simulink model "lab4"  (R2015b)
settings: Solver=ode3  StartTime=0  StopTime=30  FixedStep=Ts  RelTol=1e-3
values from neighbouring files (symbols this model uses):
  A = 12.0    (= 12)    [dev_digicomm_lab4.m]
  delta = round(310E-6*fs)    [dev_digicomm_lab4.m]
  poleN = 5    [dev_digicomm_lab4.m]
  pulsPeriod = Tb    (= 0.0003)    [dev_digicomm_lab4.m]
  pulsPhase = Tb/15    (= 2e-05)    [dev_digicomm_lab4.m]
  pulsWidth = 20    [dev_digicomm_lab4.m]
  Tb = 300E-6    (= 0.0003)    [dev_digicomm_lab4.m]
libraries: commchan3 x1, commsink2 x1, dsparch4 x1, commrandsrc2 x1, dspsigops x1
settings Model: Creator=Dennis Silage  LastModifiedBy=trejo
settings DataIOCC: SaveFormat=Array  SignalLoggingSaveFormat=ModelDataLogs
settings OptimizationCC: ExpressionDepthLimit=2147483647  InitFltsAndDblsToZero=on
settings DebuggingCC: UnderspecifiedInitializationDetection=Classic  MergeDetectMultiDrivingBlocksExec=none  SolverPrmCheckMsg=warning  FcnCallInpInsideContextMsg=UseLocalSettings  StateNameClashWarn=warning
settings HardwareCC: ProdBitPerPointer=32  ProdLargestAtomicFloat=None  ProdIntDivRoundTo=Undefined  ProdEndianess=Unspecified  ProdWordSize=32  ProdHWDeviceType=32-bit Generic
settings GRTTargetCC: GeneratePreprocessorConditionals=Disable all  CombineOutputUpdateFcns=off  GRTInterface=on
settings ConfigComp: CovModelRefEnable=Off  CovSFcnEnable=off

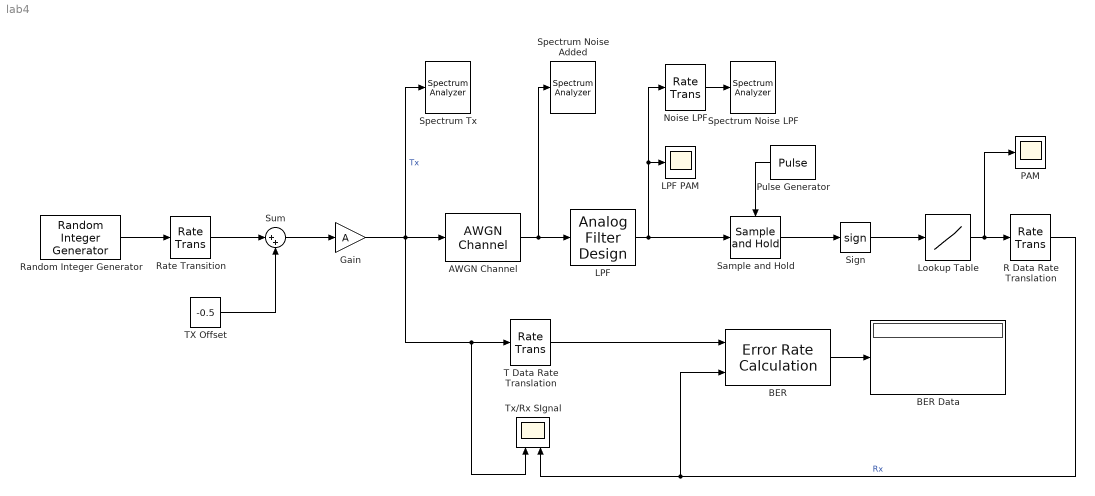
== system lab4 ==
  " PAM" : Scope
  AWGN Channel : commchan3/AWGN Channel  InputProcessing=Inherited (this choice will be removed - see release notes)  seed=randseed  noiseMode=Variance from mask  EbNodB=90  EsNodB=10  SNRdB=10  bitsPerSym=1  Ps=25  Tsym=1e-3  variance=sigma
  BER : commsink2/Error Rate Calculation  N=delta  st_delay=0  cp_mode=Entire frame  subframe=[]  PMode=Port  WsName=ErrorVec  RsMode2=off  stop=off  numErr=100  maxBits=1e6
  BER Data : Display
  Gain : Gain  Gain=A
  LPF : dsparch4/Analog Filter Design  method=Chebyshev II  filttype=Lowpass  N=poleN  Wlo=fTrad  Whi=80  Rp=2  Rs=40
  LPF PAM : Scope
  Lookup Table : Lookup  InputValues=[-1,0,1]  Table=[-A/2,-A/2,A/2]
  Noise LPF : RateTransition  OutPortSampleTime=Ts
  Pulse Generator : DiscretePulseGenerator  PulseType=Time based  Period=pulsPeriod  PulseWidth=pulsWidth  PhaseDelay=pulsPhase
  R Data Rate Translation : RateTransition  OutPortSampleTime=Ts
  Random Integer Generator : commrandsrc2/Random Integer Generator  mul=2  seed=randseed  Ts=Tb  frameBased=off  sampPerFrame=1  orient=off  outDataType=boolean
  Rate Transition : RateTransition  OutPortSampleTime=Ts
  Sample and Hold : dspsigops/Sample and Hold  trig=Rising edge  initCond=0  latchinput=off
  Sign : Signum
  Spectrum Noise Added : SpectrumAnalyzer
  Spectrum Noise LPF : SpectrumAnalyzer
  Spectrum Tx : SpectrumAnalyzer
  Sum : Sum  Inputs=|++
  T Data Rate Translation : RateTransition  OutPortSampleTime=Ts
  TX Offset : Constant  Value=-0.5
  Tx/Rx SIgnal : Scope  NumInputPorts=2
  wires:
  Random Integer Generator/1 -> Rate Transition/1
  Rate Transition/1 -> Sum/1
  TX Offset/1 -> Sum/2
  Sum/1 -> Gain/1
  Gain/1 -> Spectrum Tx/1, Tx/Rx SIgnal/1, T Data Rate Translation/1, AWGN Channel/1  "Tx"
  LPF/1 -> Sample and Hold/1, Noise LPF/1, LPF PAM/1
  Pulse Generator/1 -> Sample and Hold/Trigger
  Sample and Hold/1 -> Sign/1
  Sign/1 -> Lookup Table/1
  Lookup Table/1 -> " PAM"/1, R Data Rate Translation/1
  BER/1 -> BER Data/1
  R Data Rate Translation/1 -> BER/2, Tx/Rx SIgnal/2  "Rx"
  AWGN Channel/1 -> Spectrum Noise Added/1, LPF/1
  T Data Rate Translation/1 -> BER/1
  Noise LPF/1 -> Spectrum Noise LPF/1
